simulink model "Reglungslabor_2_Aufgabe_2_a_schaltung"  (R2023b)
settings: Solver=VariableStepAuto  StartTime=0.0  StopTime=10.0  RelTol=1e-3
values from neighbouring files (symbols this model uses):
  AB = 0.0226    [Regelungslabor_2_aufgabe_2_a_skript.m]
  c = 0.003    [Regelungslabor_2_aufgabe_2_a_skript.m]
  h = 0.1    [Regelungslabor_2_aufgabe_2_a_skript.m]
  KR = KR_array(count)    [Regelungslabor_2_aufgabe_2_a_skript.m]
  sim_time = 70    [Regelungslabor_2_aufgabe_2_a_skript.m]
settings Model: Creator=danie  LastModifiedBy=danie

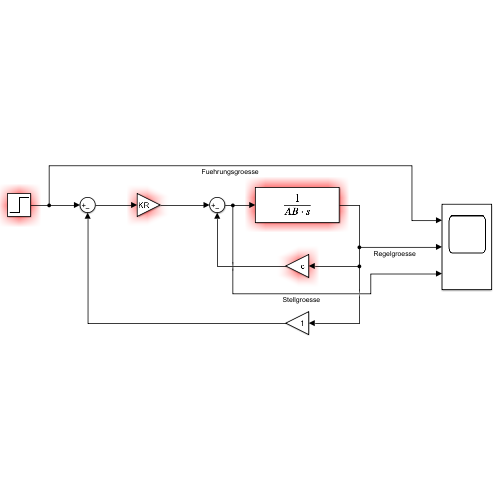
[thumbnail: Simulink's stored preview of the top-level diagram]
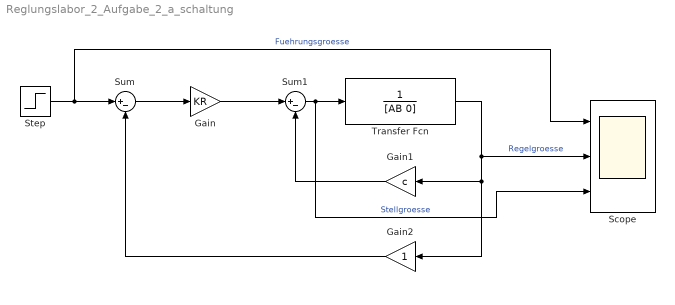
== system Reglungslabor_2_Aufgabe_2_a_schaltung ==
  Gain : Gain  Gain=KR
  Gain1 : Gain  Gain=c
  Gain2 : Gain
  Scope : Scope  NumInputPorts=3
  Step : Step  Time=sim_time  Before=h  After=0  SampleTime=0
  Sum : Sum  Inputs=|+-
  Sum1 : Sum  Inputs=|+-
  Transfer Fcn : TransferFcn  Denominator=[AB 0]
  wires:
  Sum/1 -> Gain/1
  Gain/1 -> Sum1/1
  Transfer Fcn/1 -> Scope/2, Gain2/1, Gain1/1  "Regelgroesse"
  Gain1/1 -> Sum1/2
  Gain2/1 -> Sum/2
  Step/1 -> Scope/1, Sum/1  "Fuehrungsgroesse"
  Sum1/1 -> Scope/3, Transfer Fcn/1  "Stellgroesse"
